simulink model "equation"  (R2020b)
settings: Solver=VariableStepAuto  StartTime=0.0  StopTime=10.0  RelTol=1e-3
settings Model: Creator=User  LastModifiedBy=User
settings SolverCC: AlgebraicLoopSolver=LineSearch
settings DebuggingCC: AlgebraicLoopMsg=none

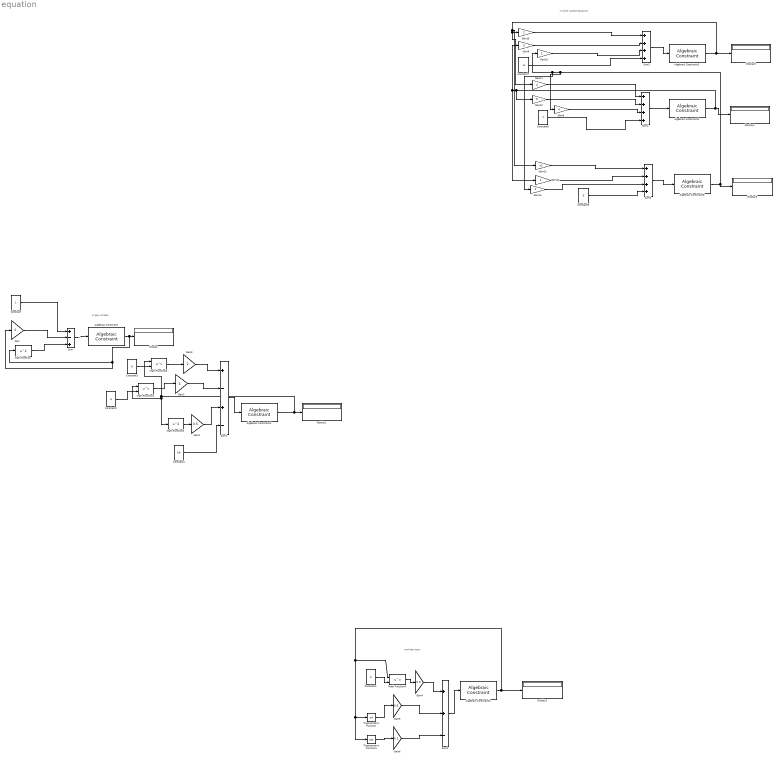
== system equation ==
  note: muliple vaiable equations
  note: nonlinear eqns
  note: single variable
  Algebraic Constraint{,1..5} (6 alike) : AlgebraicConstraint
  Constant : Constant
  Constant1 : Constant  Value=0.6
  Constant2 : Constant  Value=5
  Constant3 : Constant  Value=6
  Constant4 : Constant  Value=3
  Constant5 : Constant  Value=5
  Constant6 : Constant  Value=-7
  Constant7 : Constant  Value=-8
  Display{,1..5} (6 alike) : Display
  Gain{,3,14..15} (4 alike) : Gain  Gain=2
  Gain1 : Gain  Gain=0.5
  Gain10 : Gain  Gain=5
  Gain11 : Gain  Gain=4
  Gain12 : Gain
  Gain13 : Gain  Gain=-6
  Gain16 : Gain
  Gain2 : Gain  Gain=4
  Gain4 : Gain  Gain=0.5
  Gain5 : Gain  Gain=0.5
  Gain6 : Gain  Gain=0.1
  Gain8 : Gain  Gain=4
  Gain9 : Gain  Gain=3
  Math Function : Math  Operator=square  SaturateOnIntegerOverflow=on
  Math Function1 : Math  Operator=pow  SignedPower=on  SaturateOnIntegerOverflow=on
  Math Function2 : Math  Operator=square  SignedPower=on  OutputSignalType=real  SaturateOnIntegerOverflow=on
  Math Function3 : Math  Operator=pow  SignedPower=on  SaturateOnIntegerOverflow=on
  Math Function4 : Math  Operator=pow  SignedPower=on  SaturateOnIntegerOverflow=on
  Sum : Sum  Inputs=+-+
  Sum1 : Sum  Inputs=+-+-
  Sum2 : Sum  Inputs=++-
  Sum3 : Sum  Inputs=++++
  Sum4 : Sum  Inputs=++++
  Sum5 : Sum  Inputs=++++
  Trigonometric Function : Trigonometry
  Trigonometric Function1 : Trigonometry  Operator=cos
  wires:
  Sum/1 -> Algebraic Constraint/1
  Constant/1 -> Sum/1
  Gain/1 -> Sum/2
  Math Function/1 -> Sum/3
  Algebraic Constraint/1 -> Display/1, Math Function/1, Gain/1
  Sum1/1 -> Algebraic Constraint1/1
  Algebraic Constraint1/1 -> Math Function1/1, Math Function2/1, Math Function3/1, Display1/1
  Constant1/1 -> Sum1/4
  Gain1/1 -> Sum1/3
  Math Function2/1 -> Gain1/1
  Math Function1/1 -> Gain2/1
  Constant2/1 -> Math Function1/2
  Gain2/1 -> Sum1/2
  Math Function3/1 -> Gain3/1
  Constant3/1 -> Math Function3/2
  Gain3/1 -> Sum1/1
  Sum2/1 -> Algebraic Constraint2/1
  Gain4/1 -> Sum2/1
  Math Function4/1 -> Gain4/1
  Constant4/1 -> Math Function4/2
  Trigonometric Function/1 -> Gain5/1
  Gain5/1 -> Sum2/2
  Trigonometric Function1/1 -> Gain6/1
  Gain6/1 -> Sum2/3
  Algebraic Constraint2/1 -> Trigonometric Function1/1, Trigonometric Function/1, Math Function4/1, Display2/1
  Sum3/1 -> Algebraic Constraint3/1
  Algebraic Constraint3/1 -> Gain13/1, Gain11/1, Gain15/1, Display3/1
  Sum4/1 -> Algebraic Constraint4/1
  Algebraic Constraint5/1 -> Gain8/1, Gain14/1, Gain16/1, Display5/1
  Sum5/1 -> Algebraic Constraint5/1
  Constant6/1 -> Sum4/4
  Constant7/1 -> Sum3/4
  Constant5/1 -> Sum5/4
  Gain8/1 -> Sum4/3
  Gain10/1 -> Sum4/2
  Gain11/1 -> Sum4/1
  Gain12/1 -> Sum5/2
  Gain13/1 -> Sum5/1
  Gain14/1 -> Sum5/3
  Gain9/1 -> Sum3/2
  Gain15/1 -> Sum3/1
  Gain16/1 -> Sum3/3
  Algebraic Constraint4/1 -> Gain10/1, Gain12/1, Gain9/1, Display4/1
